simulink model "KR3_Modell"  (R2020a)
settings: Solver=VariableStepAuto  StartTime=0.0  StopTime=10.0  FixedStep=0.001  RelTol=1e-3
model workspace (MAT data in the model file):
  Damping = 0.2
  H = 2
  KR3_rbt = robotics.RigidBodyTree
  KR3_rbt.TreeInternal = robotics.manip.internal.RigidBodyTree
  KR3_rbt.TreeInternal.NumBodies = 6
  KR3_rbt.TreeInternal.Base = robotics.manip.internal.RigidBody
  KR3_rbt.TreeInternal.Base.Index = 0
  KR3_rbt.TreeInternal.Base.NameInternal = 'base'
  KR3_rbt.TreeInternal.Base.JointInternal = robotics.Joint
  KR3_rbt.TreeInternal.Base.JointInternal.Type = 'fixed'
  KR3_rbt.TreeInternal.Base.JointInternal.VelocityNumber = 0
  KR3_rbt.TreeInternal.Base.JointInternal.PositionNumber = 0
  KR3_rbt.TreeInternal.Base.JointInternal.MotionSubspace = [0; 0; 0; 0; 0; 0]
  KR3_rbt.TreeInternal.Base.JointInternal.NameInternal = 'base_jnt'
  KR3_rbt.TreeInternal.Base.ParentIndex = -1
  KR3_rbt.TreeInternal.Base.ChildrenIndices = 1
  KR3_rbt.TreeInternal.Base.MassInternal = 1
  KR3_rbt.TreeInternal.Base.CenterOfMassInternal = [0 0 0]
  KR3_rbt.TreeInternal.Base.InertiaInternal = [1  0  0; 0  1  0; 0  0  1]
  KR3_rbt.TreeInternal.Base.SpatialInertia = [1  0  0  0  0  0; 0  1  0  0  0  0; 0  0  1  0  0  0; 0  0  0  1  0  0; 0  0  0  0  1  0; 0  0  0  0  0  1]
  KR3_rbt.TreeInternal.Base.VisualsInternal{1} = robotics.manip.internal.RigidBodyGeometry
  KR3_rbt.TreeInternal.Base.VisualsInternal{1}.SourceData = {'Mesh', 'D:\Studium\SoSe21\MA_Arbeit\CAD-Dateien\baseMesh.stl'}
  KR3_rbt.TreeInternal.Base.VisualsInternal{1}.Vertices = [-0.0632426813245 -0.066875256598 -0.067146487534 -0.0603312700987 -0.0574519783258 -0.0620885789394 -0.0587106980383 -0.0573099479079 -0.052574519068 -0.0562280230224 -0.0555760525167 -0.0551131367683 ... (34239 elements, 11413x3)]
  KR3_rbt.TreeInternal.Base.VisualsInternal{1}.Faces = [1 4 7 8 8 10 11 12 13 16 16 20 ... (120618 elements, 40206x3)]
  KR3_rbt.TreeInternal.Base.CollisionsInternal = robotics.manip.internal.CollisionSet
  KR3_rbt.TreeInternal.Base.CollisionsInternal.MaxElements = 0
  KR3_rbt.TreeInternal.FastVisualizationHelper = robotics.manip.internal.FastVisualizationHelper
  KR3_rbt.TreeInternal.FastVisualizationHelper.IsUpdated = 0
  KR3_rbt.TreeInternal.FastVisualizationHelper.MeshAndFrameOptions = [0 1 1]
  KR3_rbt.TreeInternal.Gravity = [0 0 -9.80665]
  KR3_rbt.TreeInternal.Bodies{1} = robotics.manip.internal.RigidBody
  KR3_rbt.TreeInternal.Bodies{1}.Index = 1
  KR3_rbt.TreeInternal.Bodies{1}.NameInternal = 'body1'
  KR3_rbt.TreeInternal.Bodies{1}.JointInternal = robotics.Joint
  KR3_rbt.TreeInternal.Bodies{1}.JointInternal.Type = 'revolute'
  KR3_rbt.TreeInternal.Bodies{1}.JointInternal.VelocityNumber = 1
  KR3_rbt.TreeInternal.Bodies{1}.JointInternal.PositionNumber = 1
  KR3_rbt.TreeInternal.Bodies{1}.JointInternal.MotionSubspace = [0; 0; 1; 0; 0; 0]
  KR3_rbt.TreeInternal.Bodies{1}.JointInternal.InTree = 1
  KR3_rbt.TreeInternal.Bodies{1}.JointInternal.JointToParentTransform = [1  0  0  0; 0  -1  -1.22464679915e-16  0; 0  1.22464679915e-16  -1  0.183; 0  0  0  1]
  KR3_rbt.TreeInternal.Bodies{1}.JointInternal.NameInternal = 'jnt1'
  KR3_rbt.TreeInternal.Bodies{1}.JointInternal.PositionLimitsInternal = [-2.96705972839 2.96705972839]
  KR3_rbt.TreeInternal.Bodies{1}.JointInternal.JointAxisInternal = [0 0 1]
  KR3_rbt.TreeInternal.Bodies{1}.ParentIndex = 0
  KR3_rbt.TreeInternal.Bodies{1}.ChildrenIndices = [0 1]
  KR3_rbt.TreeInternal.Bodies{1}.MassInternal = 1
  KR3_rbt.TreeInternal.Bodies{1}.CenterOfMassInternal = [0 0 0]
  KR3_rbt.TreeInternal.Bodies{1}.InertiaInternal = [1  0  0; 0  1  0; 0  0  1]
  KR3_rbt.TreeInternal.Bodies{1}.SpatialInertia = [1  0  0  0  0  0; 0  1  0  0  0  0; 0  0  1  0  0  0; 0  0  0  1  0  0; 0  0  0  0  1  0; 0  0  0  0  0  1]
  KR3_rbt.TreeInternal.Bodies{1}.VisualsInternal{1} = robotics.manip.internal.RigidBodyGeometry
  KR3_rbt.TreeInternal.Bodies{1}.VisualsInternal{1}.SourceData = {'Mesh', 'D:\Studium\SoSe21\MA_Arbeit\CAD-Dateien\body1Mesh.stl'}
  KR3_rbt.TreeInternal.Bodies{1}.VisualsInternal{1}.Vertices = [0.010199774988 0.00763257872313 0.00765040656552 0.00609336374328 0.00559485983104 0.00148052396253 0.00461691664532 0.00193680962548 0.0066404142417 0.00471198977903 0.0110220154747 0.0100443195552 ... (42369 elements, 14123x3)]
  KR3_rbt.TreeInternal.Bodies{1}.VisualsInternal{1}.Faces = [1 2 3 6 5 4 4 1 2 9 7 11 ... (84738 elements, 28246x3)]
  KR3_rbt.TreeInternal.Bodies{1}.VisualsInternal{1}.Tform = [1  0  0  0; 0  -1  -1.22464679915e-16  0; 0  1.22464679915e-16  -1  0.183; 0  0  0  1]
  KR3_rbt.TreeInternal.Bodies{1}.CollisionsInternal = robotics.manip.internal.CollisionSet
  KR3_rbt.TreeInternal.Bodies{1}.CollisionsInternal.MaxElements = 0
  KR3_rbt.TreeInternal.Bodies{2} = robotics.manip.internal.RigidBody
  KR3_rbt.TreeInternal.Bodies{2}.Index = 2
  KR3_rbt.TreeInternal.Bodies{2}.NameInternal = 'body2'
  KR3_rbt.TreeInternal.Bodies{2}.JointInternal = robotics.Joint
  KR3_rbt.TreeInternal.Bodies{2}.JointInternal.Type = 'revolute'
  KR3_rbt.TreeInternal.Bodies{2}.JointInternal.VelocityNumber = 1
  KR3_rbt.TreeInternal.Bodies{2}.JointInternal.PositionNumber = 1
  KR3_rbt.TreeInternal.Bodies{2}.JointInternal.MotionSubspace = [0; 0; 1; 0; 0; 0]
  KR3_rbt.TreeInternal.Bodies{2}.JointInternal.InTree = 1
  KR3_rbt.TreeInternal.Bodies{2}.JointInternal.JointToParentTransform = [1  0  0  0.02; 0  6.12323399574e-17  -1  0; 0  1  6.12323399574e-17  -0.162; 0  0  0  1]
  KR3_rbt.TreeInternal.Bodies{2}.JointInternal.NameInternal = 'jnt2'
  KR3_rbt.TreeInternal.Bodies{2}.JointInternal.PositionLimitsInternal = [-2.96705972839 0.872664625997]
  KR3_rbt.TreeInternal.Bodies{2}.JointInternal.HomePositionInternal = -1.57079632679
  KR3_rbt.TreeInternal.Bodies{2}.JointInternal.JointAxisInternal = [0 0 1]
  KR3_rbt.TreeInternal.Bodies{2}.ParentIndex = 1
  KR3_rbt.TreeInternal.Bodies{2}.ChildrenIndices = [0 0 1]
  KR3_rbt.TreeInternal.Bodies{2}.MassInternal = 1
  KR3_rbt.TreeInternal.Bodies{2}.CenterOfMassInternal = [0 0 0]
  KR3_rbt.TreeInternal.Bodies{2}.InertiaInternal = [1  0  0; 0  1  0; 0  0  1]
  KR3_rbt.TreeInternal.Bodies{2}.SpatialInertia = [1  0  0  0  0  0; 0  1  0  0  0  0; 0  0  1  0  0  0; 0  0  0  1  0  0; 0  0  0  0  1  0; 0  0  0  0  0  1]
  KR3_rbt.TreeInternal.Bodies{2}.VisualsInternal{1} = robotics.manip.internal.RigidBodyGeometry
  KR3_rbt.TreeInternal.Bodies{2}.VisualsInternal{1}.SourceData = {'Mesh', 'D:\Studium\SoSe21\MA_Arbeit\CAD-Dateien\body2Mesh.stl'}
  KR3_rbt.TreeInternal.Bodies{2}.VisualsInternal{1}.Vertices = [0.0538231767714 0.0502161644399 0.0487190485001 0.0545652471483 0.044657304883 0.0434569939971 0.0580009557307 0.0581144578755 0.0390208996832 0.037002377212 0.0611467398703 0.0610443204641 ... (29349 elements, 9783x3)]
  KR3_rbt.TreeInternal.Bodies{2}.VisualsInternal{1}.Faces = [1 1 2 3 1 7 5 9 7 11 9 13 ... (58686 elements, 19562x3)]
  KR3_rbt.TreeInternal.Bodies{2}.VisualsInternal{1}.Tform = [6.12323399574e-17  1.83697019872e-16  1  -0.345; 1  -1.124819837e-32  -6.12323399574e-17  -0.02; 3.03535178041e-49  1  -1.83697019872e-16  4.35361937097e-17; 0  0  0  1]
  KR3_rbt.TreeInternal.Bodies{2}.CollisionsInternal = robotics.manip.internal.CollisionSet
  KR3_rbt.TreeInternal.Bodies{2}.CollisionsInternal.MaxElements = 0
  KR3_rbt.TreeInternal.Bodies{3} = robotics.manip.internal.RigidBody
  KR3_rbt.TreeInternal.Bodies{3}.Index = 3
  KR3_rbt.TreeInternal.Bodies{3}.NameInternal = 'body3'
  KR3_rbt.TreeInternal.Bodies{3}.JointInternal = robotics.Joint
  KR3_rbt.TreeInternal.Bodies{3}.JointInternal.Type = 'revolute'
  KR3_rbt.TreeInternal.Bodies{3}.JointInternal.VelocityNumber = 1
  KR3_rbt.TreeInternal.Bodies{3}.JointInternal.PositionNumber = 1
  KR3_rbt.TreeInternal.Bodies{3}.JointInternal.MotionSubspace = [0; 0; 1; 0; 0; 0]
  KR3_rbt.TreeInternal.Bodies{3}.JointInternal.InTree = 1
  KR3_rbt.TreeInternal.Bodies{3}.JointInternal.JointToParentTransform = [1  0  0  0.26; 0  1  0  0; 0  0  1  0; 0  0  0  1]
  KR3_rbt.TreeInternal.Bodies{3}.JointInternal.NameInternal = 'jnt3'
  KR3_rbt.TreeInternal.Bodies{3}.JointInternal.PositionLimitsInternal = [-1.91986217719 2.70526034059]
  KR3_rbt.TreeInternal.Bodies{3}.JointInternal.HomePositionInternal = 1.57079632679
  KR3_rbt.TreeInternal.Bodies{3}.JointInternal.JointAxisInternal = [0 0 1]
  KR3_rbt.TreeInternal.Bodies{3}.ParentIndex = 2
  KR3_rbt.TreeInternal.Bodies{3}.ChildrenIndices = [0 0 0 1]
  KR3_rbt.TreeInternal.Bodies{3}.MassInternal = 1
  KR3_rbt.TreeInternal.Bodies{3}.CenterOfMassInternal = [0 0 0]
  KR3_rbt.TreeInternal.Bodies{3}.InertiaInternal = [1  0  0; 0  1  0; 0  0  1]
  KR3_rbt.TreeInternal.Bodies{3}.SpatialInertia = [1  0  0  0  0  0; 0  1  0  0  0  0; 0  0  1  0  0  0; 0  0  0  1  0  0; 0  0  0  0  1  0; 0  0  0  0  0  1]
  KR3_rbt.TreeInternal.Bodies{3}.VisualsInternal{1} = robotics.manip.internal.RigidBodyGeometry
  KR3_rbt.TreeInternal.Bodies{3}.VisualsInternal{1}.SourceData = {'Mesh', 'D:\Studium\SoSe21\MA_Arbeit\CAD-Dateien\body3Mesh.stl'}
  KR3_rbt.TreeInternal.Bodies{3}.VisualsInternal{1}.Vertices = [0.130464464426 0.133762553334 0.129669874907 0.131500005722 0.132705897093 0.134124994278 0.133484452963 0.129170358181 0.13330963254 0.128999993205 0.134000003338 0.134547069669 ... (15924 elements, 5308x3)]
  KR3_rbt.TreeInternal.Bodies{3}.VisualsInternal{1}.Faces = [1 4 5 4 3 2 8 7 11 5 9 11 ... (31860 elements, 10620x3)]
  KR3_rbt.TreeInternal.Bodies{3}.VisualsInternal{1}.Tform = [1  0  0  -0.02; 0  -1.83697019872e-16  -1  0.605; 0  1  -1.83697019872e-16  4.35361937097e-17; 0  0  0  1]
  KR3_rbt.TreeInternal.Bodies{3}.CollisionsInternal = robotics.manip.internal.CollisionSet
  KR3_rbt.TreeInternal.Bodies{3}.CollisionsInternal.MaxElements = 0
  KR3_rbt.TreeInternal.Bodies{4} = robotics.manip.internal.RigidBody
  KR3_rbt.TreeInternal.Bodies{4}.Index = 4
  KR3_rbt.TreeInternal.Bodies{4}.NameInternal = 'body4'
  KR3_rbt.TreeInternal.Bodies{4}.JointInternal = robotics.Joint
  KR3_rbt.TreeInternal.Bodies{4}.JointInternal.Type = 'revolute'
  KR3_rbt.TreeInternal.Bodies{4}.JointInternal.VelocityNumber = 1
  KR3_rbt.TreeInternal.Bodies{4}.JointInternal.PositionNumber = 1
  KR3_rbt.TreeInternal.Bodies{4}.JointInternal.MotionSubspace = [0; 0; 1; 0; 0; 0]
  KR3_rbt.TreeInternal.Bodies{4}.JointInternal.InTree = 1
  KR3_rbt.TreeInternal.Bodies{4}.JointInternal.JointToParentTransform = [6.12323399574e-17  6.12323399574e-17  -1  0.122; -1  3.74939945665e-33  -6.12323399574e-17  -0.02; 0  1  6.12323399574e-17  0; 0  0  0  1]
  KR3_rbt.TreeInternal.Bodies{4}.JointInternal.NameInternal = 'jnt4'
  KR3_rbt.TreeInternal.Bodies{4}.JointInternal.PositionLimitsInternal = [-3.05432619099 3.05432619099]
  KR3_rbt.TreeInternal.Bodies{4}.JointInternal.JointAxisInternal = [0 0 1]
  KR3_rbt.TreeInternal.Bodies{4}.ParentIndex = 3
  KR3_rbt.TreeInternal.Bodies{4}.ChildrenIndices = [0 0 0 0 1]
  KR3_rbt.TreeInternal.Bodies{4}.MassInternal = 1
  KR3_rbt.TreeInternal.Bodies{4}.CenterOfMassInternal = [0 0 0]
  KR3_rbt.TreeInternal.Bodies{4}.InertiaInternal = [1  0  0; 0  1  0; 0  0  1]
  KR3_rbt.TreeInternal.Bodies{4}.SpatialInertia = [1  0  0  0  0  0; 0  1  0  0  0  0; 0  0  1  0  0  0; 0  0  0  1  0  0; 0  0  0  0  1  0; 0  0  0  0  0  1]
  KR3_rbt.TreeInternal.Bodies{4}.VisualsInternal{1} = robotics.manip.internal.RigidBodyGeometry
  KR3_rbt.TreeInternal.Bodies{4}.VisualsInternal{1}.SourceData = {'Mesh', 'D:\Studium\SoSe21\MA_Arbeit\CAD-Dateien\body4Mesh.stl'}
  KR3_rbt.TreeInternal.Bodies{4}.VisualsInternal{1}.Vertices = [0.2374278754 0.2374278754 0.2374278754 0.2374278754 0.237574264407 0.237607881427 0.237607881427 0.237574264407 0.237541690469 0.237541690469 0.237512126565 0.237512126565 ... (31293 elements, 10431x3)]
  KR3_rbt.TreeInternal.Bodies{4}.VisualsInternal{1}.Faces = [1 1 5 5 9 9 11 11 13 13 15 15 ... (62406 elements, 20802x3)]
  KR3_rbt.TreeInternal.Bodies{4}.VisualsInternal{1}.Tform = [6.12323399574e-17  1.83697019872e-16  1  -0.625; 6.12323399574e-17  1  -1.83697019872e-16  3.48412014357e-17; -1  6.12323399574e-17  6.12323399574e-17  0.142; 0  0  0  1]
  KR3_rbt.TreeInternal.Bodies{4}.CollisionsInternal = robotics.manip.internal.CollisionSet
  KR3_rbt.TreeInternal.Bodies{4}.CollisionsInternal.MaxElements = 0
  KR3_rbt.TreeInternal.Bodies{5} = robotics.manip.internal.RigidBody
  KR3_rbt.TreeInternal.Bodies{5}.Index = 5
  KR3_rbt.TreeInternal.Bodies{5}.NameInternal = 'body5'
  KR3_rbt.TreeInternal.Bodies{5}.JointInternal = robotics.Joint
  KR3_rbt.TreeInternal.Bodies{5}.JointInternal.Type = 'revolute'
  KR3_rbt.TreeInternal.Bodies{5}.JointInternal.VelocityNumber = 1
  KR3_rbt.TreeInternal.Bodies{5}.JointInternal.PositionNumber = 1
  KR3_rbt.TreeInternal.Bodies{5}.JointInternal.MotionSubspace = [0; 0; 1; 0; 0; 0]
  KR3_rbt.TreeInternal.Bodies{5}.JointInternal.InTree = 1
  KR3_rbt.TreeInternal.Bodies{5}.JointInternal.JointToParentTransform = [3.74939945665e-33  -1  6.12323399574e-17  0; 6.12323399574e-17  6.12323399574e-17  1  0; -1  0  6.12323399574e-17  -0.138; 0  0  0  1]
  KR3_rbt.TreeInternal.Bodies{5}.JointInternal.NameInternal = 'jnt5'
  KR3_rbt.TreeInternal.Bodies{5}.JointInternal.PositionLimitsInternal = [-2.09439510239 2.09439510239]
  KR3_rbt.TreeInternal.Bodies{5}.JointInternal.JointAxisInternal = [0 0 1]
  KR3_rbt.TreeInternal.Bodies{5}.ParentIndex = 4
  KR3_rbt.TreeInternal.Bodies{5}.ChildrenIndices = [0 0 0 0 0 1]
  KR3_rbt.TreeInternal.Bodies{5}.MassInternal = 1
  KR3_rbt.TreeInternal.Bodies{5}.CenterOfMassInternal = [0 0 0]
  KR3_rbt.TreeInternal.Bodies{5}.InertiaInternal = [1  0  0; 0  1  0; 0  0  1]
  KR3_rbt.TreeInternal.Bodies{5}.SpatialInertia = [1  0  0  0  0  0; 0  1  0  0  0  0; 0  0  1  0  0  0; 0  0  0  1  0  0; 0  0  0  0  1  0; 0  0  0  0  0  1]
  KR3_rbt.TreeInternal.Bodies{5}.VisualsInternal{1} = robotics.manip.internal.RigidBodyGeometry
  KR3_rbt.TreeInternal.Bodies{5}.VisualsInternal{1}.SourceData = {'Mesh', 'D:\Studium\SoSe21\MA_Arbeit\CAD-Dateien\body5Mesh.stl'}
  KR3_rbt.TreeInternal.Bodies{5}.VisualsInternal{1}.Vertices = [0.280791640282 0.280418545008 0.280028581619 0.281197071075 0.280991524458 0.281554192305 0.280000001192 0.280000001192 0.281901538372 0.281152635813 0.28150805831 0.280768126249 ... (183075 elements, 61025x3)]
  KR3_rbt.TreeInternal.Bodies{5}.VisualsInternal{1}.Faces = [1 4 6 2 3 2 5 9 11 13 10 14 ... (366135 elements, 122045x3)]
  KR3_rbt.TreeInternal.Bodies{5}.VisualsInternal{1}.Tform = [1  -7.49879891331e-33  -6.12323399574e-17  -0.28; -6.12323399574e-17  -1.22464679915e-16  -1  0.625; 4.82715273077e-33  1  -1.22464679915e-16  1.37160441505e-17; 0  0  0  1]
  KR3_rbt.TreeInternal.Bodies{5}.CollisionsInternal = robotics.manip.internal.CollisionSet
  KR3_rbt.TreeInternal.Bodies{5}.CollisionsInternal.MaxElements = 0
  KR3_rbt.TreeInternal.Bodies{6} = robotics.manip.internal.RigidBody
  KR3_rbt.TreeInternal.Bodies{6}.Index = 6
  KR3_rbt.TreeInternal.Bodies{6}.NameInternal = 'body6'
  KR3_rbt.TreeInternal.Bodies{6}.JointInternal = robotics.Joint
  KR3_rbt.TreeInternal.Bodies{6}.JointInternal.Type = 'revolute'
  KR3_rbt.TreeInternal.Bodies{6}.JointInternal.VelocityNumber = 1
  KR3_rbt.TreeInternal.Bodies{6}.JointInternal.PositionNumber = 1
  KR3_rbt.TreeInternal.Bodies{6}.JointInternal.MotionSubspace = [0; 0; 1; 0; 0; 0]
  KR3_rbt.TreeInternal.Bodies{6}.JointInternal.InTree = 1
  KR3_rbt.TreeInternal.Bodies{6}.JointInternal.JointToParentTransform = [6.12323399574e-17  6.12323399574e-17  -1  0.075; -1  3.74939945665e-33  -6.12323399574e-17  0; 0  1  6.12323399574e-17  0; 0  0  0  1]
  KR3_rbt.TreeInternal.Bodies{6}.JointInternal.NameInternal = 'jnt6'
  KR3_rbt.TreeInternal.Bodies{6}.JointInternal.PositionLimitsInternal = [-6.10865238198 6.10865238198]
  KR3_rbt.TreeInternal.Bodies{6}.JointInternal.JointAxisInternal = [0 0 1]
  KR3_rbt.TreeInternal.Bodies{6}.ParentIndex = 5
  KR3_rbt.TreeInternal.Bodies{6}.ChildrenIndices = [0 0 0 0 0]
  KR3_rbt.TreeInternal.Bodies{6}.MassInternal = 1
  KR3_rbt.TreeInternal.Bodies{6}.CenterOfMassInternal = [0 0 0]
  KR3_rbt.TreeInternal.Bodies{6}.InertiaInternal = [1  0  0; 0  1  0; 0  0  1]
  KR3_rbt.TreeInternal.Bodies{6}.SpatialInertia = [1  0  0  0  0  0; 0  1  0  0  0  0; 0  0  1  0  0  0; 0  0  0  1  0  0; 0  0  0  0  1  0; 0  0  0  0  0  1]
  KR3_rbt.TreeInternal.Bodies{6}.VisualsInternal{1} = robotics.manip.internal.RigidBodyGeometry
  KR3_rbt.TreeInternal.Bodies{6}.VisualsInternal{1}.SourceData = {'Mesh', 'D:\Studium\SoSe21\MA_Arbeit\CAD-Dateien\body6Mesh.stl'}
  KR3_rbt.TreeInternal.Bodies{6}.VisualsInternal{1}.Vertices = [0.338999986649 0.338999986649 0.338999986649 0.338999986649 0.338999986649 0.338999986649 0.338999986649 0.338999986649 0.338999986649 0.338999986649 0.338999986649 0.338999986649 ... (7587 elements, 2529x3)]
  KR3_rbt.TreeInternal.Bodies{6}.VisualsInternal{1}.Faces = [1 4 4 6 7 8 8 10 11 11 13 14 ... (15174 elements, 5058x3)]
  KR3_rbt.TreeInternal.Bodies{6}.VisualsInternal{1}.Tform = [1.22464679915e-16  1.22464679915e-16  1  -0.625; 6.12323399574e-17  1  -1.22464679915e-16  -8.02143653442e-18; -1  6.12323399574e-17  1.22464679915e-16  0.355; 0  0  0  1]
  KR3_rbt.TreeInternal.Bodies{6}.CollisionsInternal = robotics.manip.internal.CollisionSet
  KR3_rbt.TreeInternal.Bodies{6}.CollisionsInternal.MaxElements = 0
  KR3_rbt.TreeInternal.NumNonFixedBodies = 6
  KR3_rbt.TreeInternal.PositionNumber = 6
  KR3_rbt.TreeInternal.VelocityNumber = 6
  KR3_rbt.TreeInternal.PositionDoFMap = [1  1; 2  2; 3  3; 4  4; 5  5; 6  6]
  KR3_rbt.TreeInternal.VelocityDoFMap = [1  1; 2  2; 3  3; 4  4; 5  5; 6  6]
  KR3_rbt.TreeInternal.MaxNumBodies = 6
  KR3_rbt.TreeInternal.MaxNameLength = 200
  KR3_rbt.TreeInternal.MaxJointPositionNumber = 7
  KR3_rbt.TreeInternal.VisualizationInfo = robotics.manip.internal.VisualizationInfo
  KR3_rbt.TreeInternal.VisualizationInfo.ShowTag = 'DO_NOT_EDIT_41EHK'
  KR3_rbt.TreeInternal.DataFormatInternal = 'column'
  L = 20
  W = 2
  den = 1110
  initTargetPose = [0.264 0 0.61 -0.471238898038 1.32645023152 -0.418879020479]
  rho = 1000
  st = 0.04
  tol = 0.01
values from neighbouring files (symbols this model uses):
  s = char(posmsg{k})    [Messbahn_Quadrat.m]
  traj = [traj, axis_conf]    [generate_trajectory.m]
undefined symbols (not defined in the file or in its folder): X, Y, Z
libraries: sm_lib x33, nesl_utility x17, fl_ps_legacy_lib x12, simulink x1
settings Model: OrderedModelArguments=off  Creator=Arbeit  LastModifiedBy=Arbeit
settings DataIOCC: ReturnWorkspaceOutputs=off
settings DebuggingCC: ArithmeticOperatorsInVariantConditions=warning
settings SFSimCC: SimUseLocalCustomCode=off  CustomCodeUndefinedFunction=UseInterfaceOnly
settings RTWCC: RTWUseLocalCustomCode=off

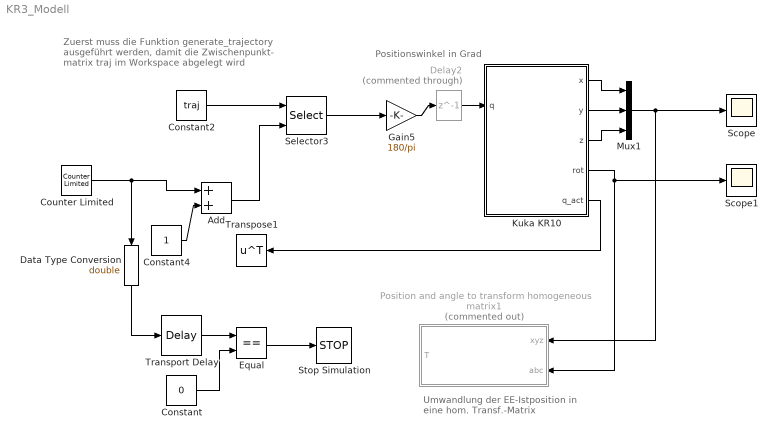
== system KR3_Modell ==
  note: Zuerst muss die Funktion generate_trajectory
      | ausgeführt werden, damit die Zwischenpunkt-
      | matrix traj im Workspace abgelegt wird
  note: Positionswinkel in Grad
  note: Umwandlung der EE-Istposition in eine hom. Transf.-Matrix
  Add : Sum
  Constant : Constant  Value=0
  Constant2 : Constant  Value=traj
  Constant4 : Constant
  Counter Limited : simulink/Sources/Counter Limited  uplimit=size(traj,2)-1  tsamp=-1
  Data Type Conversion : DataTypeConversion  OutDataTypeStr=double
  Delay2 : Delay  Commented=through  DelayLength=1
  Equal : RelationalOperator  Operator===  OutDataTypeStr=boolean  RndMeth=Simplest
  Gain5 : Gain  Gain=180/pi
  Kuka KR10 : Subsystem
      mask Display: image('kuka_kr10_r1100.jpg');
  Mux1 : Mux  Inputs=3
  Position and angle to transform homogeneous matrix1 : MATLAB Function  Commented=on  TreatAsAtomicUnit=on
  Scope : Scope
  Scope1 : Scope
  Selector3 : Selector  NumberOfDimensions=2  InputPortWidth=3  IndexOptions=Select all,Starting index (port)  Indices=[1 3],1  OutputSizes=1,1
  Stop Simulation : Stop
  Transport Delay : TransportDelay  InitialOutput=1
  Transpose1 : Math  Operator=transpose  SaturateOnIntegerOverflow=on
  wires:
  Kuka KR10/2(y) -> Mux1/2
  Kuka KR10/1(x) -> Mux1/1
  Kuka KR10/3(z) -> Mux1/3
  Kuka KR10/4(rot) -> Position and angle to transform homogeneous matrix1/2(abc), Scope1/1
  Mux1/1 -> Position and angle to transform homogeneous matrix1/1(xyz), Scope/1
  Constant2/1 -> Selector3/1
  Selector3/1 -> Gain5/1
  Gain5/1 -> Delay2/1
  Delay2/1 -> Kuka KR10/1(q)
  Kuka KR10/5(q_act) -> Transpose1/1
  Counter Limited/1 -> Add/1, Data Type Conversion/1
  Add/1 -> Selector3/2
  Constant4/1 -> Add/2
  Transport Delay/1 -> Equal/1
  Constant/1 -> Equal/2
  Equal/1 -> Stop Simulation/1
  Data Type Conversion/1 -> Transport Delay/1

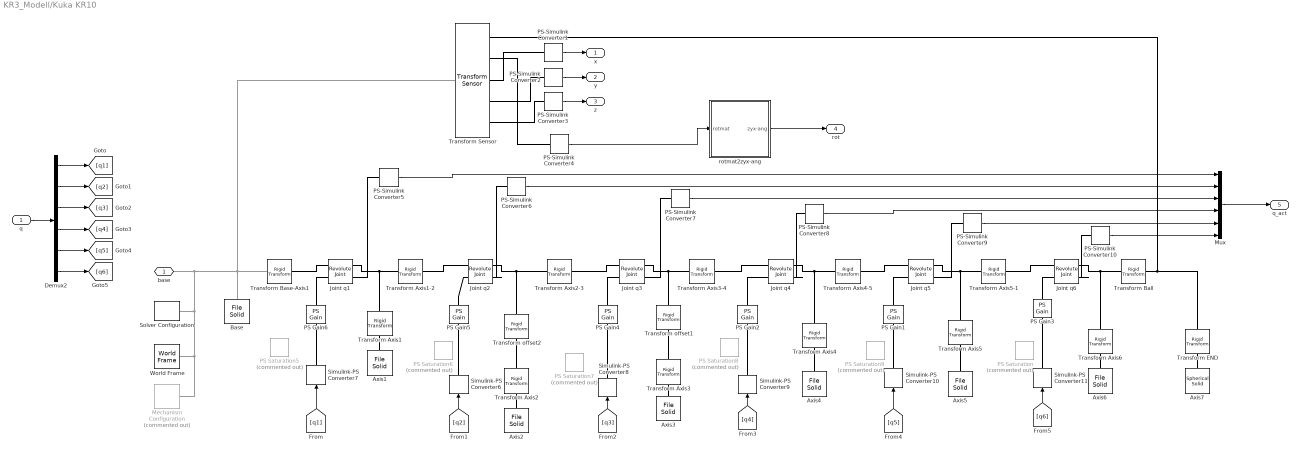
== system KR3_Modell/Kuka KR10 ==
  q : Inport
   Joint q{1..6} (6 alike) : sm_lib/Joints/Revolute Joint  JointMode=Normal  SenseConstraintForce=off  SenseConstraintForceX=off  SenseConstraintForceY=off  SenseConstraintForceZ=off  SenseConstraintTorque=off  SenseConstraintTorqueX=off  SenseConstraintTorqueY=off  SenseConstraintTorqueZ=off  SenseTotalForce=off  SenseTotalForceX=off  SenseTotalForceY=off  SenseTotalForceZ=off  SenseTotalTorque=off  SenseTotalTorqueX=off  SenseTotalTorqueY=off  SenseTotalTorqueZ=off  CompositeWrenchDir=FollowerOnBase  CompositeWrenchFrame=BaseFrame  EquilibriumPosition=0  EquilibriumPositionUnits=deg  SpringStiffness=0  SpringStiffnessUnits=N*m/deg  DampingCoefficient=0  DampingCoefficientUnits=N*m/(deg/s)  TorqueActuationMode=ComputedTorque  MotionActuationMode=InputMotion  SensePosition=on  SenseVelocity=off  SenseAcceleration=off  SenseTorqueForce=off  SenseLowerLimitTorqueForce=off  SenseUpperLimitTorqueForce=off  LowerLimitSpecify=off  LowerLimitBound=-90  LowerLimitBoundUnits=deg  LowerLimitStiffness=1e4  LowerLimitStiffnessUnits=N*m/deg  LowerLimitDamping=10  LowerLimitDampingUnits=N*m/(deg/s)  LowerLimitTransitionRegionWidth=0.1  LowerLimitTransitionRegionWidthUnits=deg  UpperLimitSpecify=off  UpperLimitBound=90  UpperLimitBoundUnits=deg  UpperLimitStiffness=1e4  UpperLimitStiffnessUnits=N*m/deg  UpperLimitDamping=10  UpperLimitDampingUnits=N*m/(deg/s)  UpperLimitTransitionRegionWidth=0.1  UpperLimitTransitionRegionWidthUnits=deg  PositionTargetSpecify=on  PositionTargetPriority=Low  PositionTargetValue=0  PositionTargetValueUnits=deg  VelocityTargetSpecify=off  VelocityTargetPriority=High  VelocityTargetValue=0  VelocityTargetValueUnits=deg/s
  Axis1 : sm_lib/Body Elements/File Solid  ExtGeomFileName=D:\Studium\SoSe21\MA_Arbeit\CAD-Dateien\body1Test.step  UnitType=FromFile  ExtGeomFileUnits=m  StepReaderType=OCC  ExportConvexHullGeometry=off  InertiaType=CalculateFromGeometry  Mass=1  MassUnits=kg  CenterOfMass=[0 0 0]  CenterOfMassUnits=m  MomentsOfInertia=[1 1 1]  MomentsOfInertiaUnits=kg*m^2  ProductsOfInertia=[1 1 1]  ProductsOfInertiaUnits=kg*m^2  BasedOnType=Density  Density=den  DensityUnits=kg/m^3  DoExposeReferenceFrame=on  SerializedFrames=<Frames/>  GraphicType=FromGeometry  MarkerShape=Sphere  MarkerSize=10  GraphicVisPropType=SimpleVisualProperties  GraphicDiffuseColor=[1 0.39 0]  GraphicSpecularColor=[0.5 0.5 0.5 1.0]  GraphicAmbientColor=[0.15 0.15 0.15 1.0]  GraphicEmissiveColor=[0.0 0.0 0.0 1.0]  GraphicShininess=75  GraphicOpacity=1
  Axis2 : sm_lib/Body Elements/File Solid  ExtGeomFileName=D:\Studium\SoSe21\MA_Arbeit\CAD-Dateien\body2Test.step  UnitType=FromFile  ExtGeomFileUnits=m  StepReaderType=OCC  ExportConvexHullGeometry=off  InertiaType=CalculateFromGeometry  Mass=1  MassUnits=kg  CenterOfMass=[0 0 0]  CenterOfMassUnits=m  MomentsOfInertia=[1 1 1]  MomentsOfInertiaUnits=kg*m^2  ProductsOfInertia=[1 1 1]  ProductsOfInertiaUnits=kg*m^2  BasedOnType=Density  Density=den  DensityUnits=kg/m^3  DoExposeReferenceFrame=on  SerializedFrames=<Frames/>  GraphicType=FromGeometry  MarkerShape=Sphere  MarkerSize=10  GraphicVisPropType=SimpleVisualProperties  GraphicDiffuseColor=[1 0.39 0]  GraphicSpecularColor=[0.5 0.5 0.5 1.0]  GraphicAmbientColor=[0.15 0.15 0.15 1.0]  GraphicEmissiveColor=[0.0 0.0 0.0 1.0]  GraphicShininess=75  GraphicOpacity=1
  Axis3 : sm_lib/Body Elements/File Solid  ExtGeomFileName=D:\Studium\SoSe21\MA_Arbeit\CAD-Dateien\body3Test.step  UnitType=FromFile  ExtGeomFileUnits=m  StepReaderType=OCC  ExportConvexHullGeometry=off  InertiaType=CalculateFromGeometry  Mass=1  MassUnits=kg  CenterOfMass=[0 0 0]  CenterOfMassUnits=m  MomentsOfInertia=[1 1 1]  MomentsOfInertiaUnits=kg*m^2  ProductsOfInertia=[1 1 1]  ProductsOfInertiaUnits=kg*m^2  BasedOnType=Density  Density=den  DensityUnits=kg/m^3  DoExposeReferenceFrame=on  SerializedFrames=<Frames/>  GraphicType=FromGeometry  MarkerShape=Sphere  MarkerSize=10  GraphicVisPropType=SimpleVisualProperties  GraphicDiffuseColor=[1 0.39 0]  GraphicSpecularColor=[0.5 0.5 0.5 1.0]  GraphicAmbientColor=[0.15 0.15 0.15 1.0]  GraphicEmissiveColor=[0.0 0.0 0.0 1.0]  GraphicShininess=75  GraphicOpacity=1
  Axis4 : sm_lib/Body Elements/File Solid  ExtGeomFileName=D:\Studium\SoSe21\MA_Arbeit\CAD-Dateien\body4Test.step  UnitType=FromFile  ExtGeomFileUnits=m  StepReaderType=OCC  ExportConvexHullGeometry=off  InertiaType=CalculateFromGeometry  Mass=1  MassUnits=kg  CenterOfMass=[0 0 0]  CenterOfMassUnits=m  MomentsOfInertia=[1 1 1]  MomentsOfInertiaUnits=kg*m^2  ProductsOfInertia=[1 1 1]  ProductsOfInertiaUnits=kg*m^2  BasedOnType=Density  Density=den  DensityUnits=kg/m^3  DoExposeReferenceFrame=on  SerializedFrames=<Frames/>  GraphicType=FromGeometry  MarkerShape=Sphere  MarkerSize=10  GraphicVisPropType=SimpleVisualProperties  GraphicDiffuseColor=[1 0.39 0]  GraphicSpecularColor=[0.5 0.5 0.5 1.0]  GraphicAmbientColor=[0.15 0.15 0.15 1.0]  GraphicEmissiveColor=[0.0 0.0 0.0 1.0]  GraphicShininess=75  GraphicOpacity=1
  Axis5 : sm_lib/Body Elements/File Solid  ExtGeomFileName=D:\Studium\SoSe21\MA_Arbeit\CAD-Dateien\body5Test.step  UnitType=FromFile  ExtGeomFileUnits=m  StepReaderType=OCC  ExportConvexHullGeometry=off  InertiaType=CalculateFromGeometry  Mass=1  MassUnits=kg  CenterOfMass=[0 0 0]  CenterOfMassUnits=m  MomentsOfInertia=[1 1 1]  MomentsOfInertiaUnits=kg*m^2  ProductsOfInertia=[1 1 1]  ProductsOfInertiaUnits=kg*m^2  BasedOnType=Density  Density=den  DensityUnits=kg/m^3  DoExposeReferenceFrame=on  SerializedFrames=<Frames/>  GraphicType=FromGeometry  MarkerShape=Sphere  MarkerSize=10  GraphicVisPropType=SimpleVisualProperties  GraphicDiffuseColor=[1 0.39 0]  GraphicSpecularColor=[0.5 0.5 0.5 1.0]  GraphicAmbientColor=[0.15 0.15 0.15 1.0]  GraphicEmissiveColor=[0.0 0.0 0.0 1.0]  GraphicShininess=75  GraphicOpacity=1
  Axis6 : sm_lib/Body Elements/File Solid  ExtGeomFileName=D:\Studium\SoSe21\MA_Arbeit\CAD-Dateien\body6Test.step  UnitType=FromFile  ExtGeomFileUnits=m  StepReaderType=OCC  ExportConvexHullGeometry=off  InertiaType=CalculateFromGeometry  Mass=1  MassUnits=kg  CenterOfMass=[0 0 0]  CenterOfMassUnits=m  MomentsOfInertia=[1 1 1]  MomentsOfInertiaUnits=kg*m^2  ProductsOfInertia=[1 1 1]  ProductsOfInertiaUnits=kg*m^2  BasedOnType=Density  Density=den  DensityUnits=kg/m^3  DoExposeReferenceFrame=on  SerializedFrames=<Frames/>  GraphicType=FromGeometry  MarkerShape=Sphere  MarkerSize=10  GraphicVisPropType=SimpleVisualProperties  GraphicDiffuseColor=[.2 .2 .2]  GraphicSpecularColor=[0.5 0.5 0.5 1.0]  GraphicAmbientColor=[0.15 0.15 0.15 1.0]  GraphicEmissiveColor=[0.0 0.0 0.0 1.0]  GraphicShininess=75  GraphicOpacity=1
  Axis7 : sm_lib/Body Elements/Spherical Solid  GraphicAmbientColor=[0.15 0.15 0.15 1.0]  BasedOnType=Mass  CenterOfMass=[0 0 0]  CenterOfMassUnits=m  GraphicDiffuseColor=[1 1 1]  Density=den  DensityUnits=kg/m^3  DoExposeReferenceFrame=on  GraphicEmissiveColor=[0.0 0.0 0.0 1.0]  ExportEntireGeometry=off  SerializedExposedGeometries=<ExposedGeometries/>  SerializedFrames=<Frames/>  MarkerShape=Sphere  MarkerSize=10  GraphicType=FromGeometry  InertiaType=CalculateFromGeometry  Mass=0.254  MassUnits=kg  MomentsOfInertia=[1 1 1]  MomentsOfInertiaUnits=kg*m^2  GraphicOpacity=1  ProductsOfInertia=[1 1 1]  ProductsOfInertiaUnits=kg*m^2  GraphicShininess=75  GraphicSpecularColor=[0.5 0.5 0.5 1.0]  SphereRadius=0.034  SphereRadiusUnits=m  GraphicVisPropType=SimpleVisualProperties
  Base : sm_lib/Body Elements/File Solid  ExtGeomFileName=D:\Studium\SoSe21\MA_Arbeit\CAD-Dateien\baseTest.step  UnitType=FromFile  ExtGeomFileUnits=m  StepReaderType=OCC  ExportConvexHullGeometry=off  InertiaType=CalculateFromGeometry  Mass=1  MassUnits=kg  CenterOfMass=[0 0 0]  CenterOfMassUnits=m  MomentsOfInertia=[1 1 1]  MomentsOfInertiaUnits=kg*m^2  ProductsOfInertia=[1 1 1]  ProductsOfInertiaUnits=kg*m^2  BasedOnType=Density  Density=den  DensityUnits=kg/m^3  DoExposeReferenceFrame=on  SerializedFrames=<Frames/>  GraphicType=FromGeometry  MarkerShape=Sphere  MarkerSize=10  GraphicVisPropType=SimpleVisualProperties  GraphicDiffuseColor=[.2 .2 .2]  GraphicSpecularColor=[0.5 0.5 0.5 1.0]  GraphicAmbientColor=[0.15 0.15 0.15 1.0]  GraphicEmissiveColor=[0.0 0.0 0.0 1.0]  GraphicShininess=75  GraphicOpacity=1
  Demux2 : Demux  Outputs=6
  Mechanism Configuration : sm_lib/Utilities/Mechanism Configuration  Commented=on  UniformGravity=Constant  GravityVector=[0 0 -9.80665]  GravityVectorUnits=m/s^2  GravityUnits=m/s^2  LinearizationDelta=0.001  JointModeTransitionNonlinearIterations=2
  Mux : Mux  Inputs=6
  PS Gain{1..6} (6 alike) : fl_ps_legacy_lib/Legacy Physical Signals/Functions/PS Gain  gain=pi/180
  PS Saturation : fl_ps_legacy_lib/Legacy Physical Signals/Nonlinear Operators/PS Saturation  Commented=on  upper_limit=350  lower_limit=-350
      settings: SourceProductBaseCode=SS  InternalSimscapePortConfiguration="{\"Bottom\":[],\"Left\":[{\"id\":\"I\",\"label\":\"\",\"type\":\"input\"}],\"Right\":[{\"id\":\"O\",\"label\":\"\",\"type\":\"output\"}],\"Top\":[]}"
  PS Saturation5 : fl_ps_legacy_lib/Legacy Physical Signals/Nonlinear Operators/PS Saturation  Commented=on  upper_limit=170  lower_limit=-170
      settings: SourceProductBaseCode=SS  InternalSimscapePortConfiguration="{\"Bottom\":[],\"Left\":[{\"id\":\"I\",\"label\":\"\",\"type\":\"input\"}],\"Right\":[{\"id\":\"O\",\"label\":\"\",\"type\":\"output\"}],\"Top\":[]}"
  PS Saturation6 : fl_ps_legacy_lib/Legacy Physical Signals/Nonlinear Operators/PS Saturation  Commented=on  upper_limit=50  lower_limit=-170
      settings: SourceProductBaseCode=SS  InternalSimscapePortConfiguration="{\"Bottom\":[],\"Left\":[{\"id\":\"I\",\"label\":\"\",\"type\":\"input\"}],\"Right\":[{\"id\":\"O\",\"label\":\"\",\"type\":\"output\"}],\"Top\":[]}"
  PS Saturation7 : fl_ps_legacy_lib/Legacy Physical Signals/Nonlinear Operators/PS Saturation  Commented=on  upper_limit=155  lower_limit=-110
      settings: SourceProductBaseCode=SS  InternalSimscapePortConfiguration="{\"Bottom\":[],\"Left\":[{\"id\":\"I\",\"label\":\"\",\"type\":\"input\"}],\"Right\":[{\"id\":\"O\",\"label\":\"\",\"type\":\"output\"}],\"Top\":[]}"
  PS Saturation8 : fl_ps_legacy_lib/Legacy Physical Signals/Nonlinear Operators/PS Saturation  Commented=on  upper_limit=175  lower_limit=-175
      settings: SourceProductBaseCode=SS  InternalSimscapePortConfiguration="{\"Bottom\":[],\"Left\":[{\"id\":\"I\",\"label\":\"\",\"type\":\"input\"}],\"Right\":[{\"id\":\"O\",\"label\":\"\",\"type\":\"output\"}],\"Top\":[]}"
  PS Saturation9 : fl_ps_legacy_lib/Legacy Physical Signals/Nonlinear Operators/PS Saturation  Commented=on  upper_limit=120  lower_limit=-120
      settings: SourceProductBaseCode=SS  InternalSimscapePortConfiguration="{\"Bottom\":[],\"Left\":[{\"id\":\"I\",\"label\":\"\",\"type\":\"input\"}],\"Right\":[{\"id\":\"O\",\"label\":\"\",\"type\":\"output\"}],\"Top\":[]}"
  PS-Simulink Converter{1..10} (10 alike) : nesl_utility/PS-Simulink Converter  PhysicalDomain=network_engine_domain  SubClassName=ps_output  LeftPortType=input  RightPortType=output  PseudoPeriodic=off  Frequencies=[]  Unit=1  AffineConversion=off
      settings: SourceProductBaseCode=PW,SS
  Simulink-PS Converter{6..11} (6 alike) : nesl_utility/Simulink-PS Converter  PhysicalDomain=network_engine_domain  SubClassName=ps_input  LeftPortType=input  RightPortType=output  PseudoPeriodic=off  Frequencies=[]  NoiseDistribution=none  NoiseParameters=[]  Unit=1  AffineConversion=off  FilteringAndDerivatives=provide  SimscapeFilterOrder=1  InputFilterTimeConstant=0.001  UdotUserProvided=0
      settings: SourceProductBaseCode=PW,SS
  Solver Configuration : nesl_utility/Solver Configuration  PhysicalDomain=network_engine_domain  SubClassName=solver  LeftPortType=input  RightPortType=generic  Tones=[]  Harmonics=[]  SimulateNoise=off  Profile=off  UseLocalSampling=off  EnableSwitchedLinearOptims=on  FrequencyDomain=off  UseCCode=off  RelTol=0.001  AbsTol=1e-06  MinStep=1e-09  ToWorkspace=off  RevertToSquareIcSolve=off  NumHomotopyIterations=100  PhasorMode=off  PhasorModeNumHarmonics=1  DoDC=off  ResidualTolerance=1e-04  UseLocalSolver=on  LocalSolverChoice=NE_BACKWARD_EULER_ADVANCER  LocalSolverSampleTime=0.01  DoFixedCost=on  MaxNonlinIter=3  MaxModeIter=2  ComputeImpulses=off  ImpulseIterations=2  LinearAlgebra=auto  EquationFormulation=NE_TIME_EF  DelaysMemoryBudget=1024  AutomaticFiltering=on  FilteringTimeConstant=0.001  PartitionStorageMethod=AS_NEEDED  PartitionMemoryBudget=1024  PartitionMethod=FAST
      settings: SourceProductBaseCode=PW,SS
  Transform Sensor : sm_lib/Frames and Transforms/Transform Sensor  MeasurementFrame=World  SenseAngle=off  SenseAxis=off  SenseAngle1=off  SenseAngle2=off  SenseAngle3=off  SenseQ=off  SenseR=on  SenseOmegaX=off  SenseOmegaY=off  SenseOmegaZ=off  SenseOmega1=off  SenseOmega2=off  SenseOmega3=off  SenseQDot=off  SenseRDot=off  SenseAlphaX=off  SenseAlphaY=off  SenseAlphaZ=off  SenseAlpha1=off  SenseAlpha2=off  SenseAlpha3=off  SenseQDDot=off  SenseRDDot=off  SenseX=on  SenseY=on  SenseZ=on  SenseRad=off  SenseAzim=off  SenseDist=off  SenseInc=off  SenseXDot=off  SenseYDot=off  SenseZDot=off  SenseRadDot=off  SenseAzimDot=off  SenseDistDot=off  SenseIncDot=off  SenseXDDot=off  SenseYDDot=off  SenseZDDot=off  SenseRadDDot=off  SenseAzimDDot=off  SenseDistDDot=off  SenseIncDDot=off
  Transform Axis1 : sm_lib/Frames and Transforms/Rigid Transform  TranslationMethod=Cartesian  TranslationStandardOffset=0  TranslationLengthUnit=mm  TranslationStandardAxis=+Z  TranslationCartesianOffset=[0 0 183]  TranslationROffset=0  TranslationROffsetUnits=m  TranslationZOffset=0  TranslationZOffsetUnits=m  TranslationThetaOffset=0  TranslationThetaOffsetUnits=deg  RotationMethod=RotationSequence  RotationAngleUnits=deg  RotationStandardAxis=+Z  RotationAngle=0.0  RotationArbitraryAxis=[0 0 1]  FollAlignAxisA=+Z  BaseAlignAxisA=+Z  FollAlignAxisB=+X  BaseAlignAxisB=+X  RotationSequenceAxes=FollowerAxes  RotationSequence=ZYX  RotationSequenceAngles=[0 0 pi]  RotationSequenceAnglesUnits=rad  RotationMatrix=[1 0 0; 0 1 0; 0 0 1]
  Transform Axis1-2 : sm_lib/Frames and Transforms/Rigid Transform  TranslationMethod=Cartesian  TranslationStandardOffset=0  TranslationLengthUnit=mm  TranslationStandardAxis=+Z  TranslationCartesianOffset=[20 0 -162]  TranslationROffset=0  TranslationROffsetUnits=m  TranslationZOffset=0  TranslationZOffsetUnits=m  TranslationThetaOffset=0  TranslationThetaOffsetUnits=deg  RotationMethod=RotationSequence  RotationAngleUnits=deg  RotationStandardAxis=+Z  RotationAngle=0.0  RotationArbitraryAxis=[0 0 1]  FollAlignAxisA=+X  BaseAlignAxisA=+X  FollAlignAxisB=+Z  BaseAlignAxisB=-Y  RotationSequenceAxes=FollowerAxes  RotationSequence=ZYX  RotationSequenceAngles=[0 0 pi/2]  RotationSequenceAnglesUnits=rad  RotationMatrix=[1 0 0; 0 1 0; 0 0 1]
  Transform Axis2 : sm_lib/Frames and Transforms/Rigid Transform  TranslationMethod=Cartesian  TranslationStandardOffset=0  TranslationLengthUnit=mm  TranslationStandardAxis=+Z  TranslationCartesianOffset=[20 0 345]  TranslationROffset=0  TranslationROffsetUnits=m  TranslationZOffset=0  TranslationZOffsetUnits=m  TranslationThetaOffset=0  TranslationThetaOffsetUnits=deg  RotationMethod=RotationSequence  RotationAngleUnits=deg  RotationStandardAxis=-X  RotationAngle=90  RotationArbitraryAxis=[0 0 1]  FollAlignAxisA=+Z  BaseAlignAxisA=-Y  FollAlignAxisB=+X  BaseAlignAxisB=+X  RotationSequenceAxes=FollowerAxes  RotationSequence=ZYX  RotationSequenceAngles=[0 0 -90]  RotationSequenceAnglesUnits=deg  RotationMatrix=[1 0 0; 0 1 0; 0 0 1]
  Transform Axis2-3 : sm_lib/Frames and Transforms/Rigid Transform  TranslationMethod=Cartesian  TranslationStandardOffset=0  TranslationLengthUnit=mm  TranslationStandardAxis=+Z  TranslationCartesianOffset=[260 0 0]  TranslationROffset=0  TranslationROffsetUnits=m  TranslationZOffset=0  TranslationZOffsetUnits=m  TranslationThetaOffset=0  TranslationThetaOffsetUnits=deg  RotationMethod=RotationSequence  RotationAngleUnits=deg  RotationStandardAxis=+Z  RotationAngle=0.0  RotationArbitraryAxis=[0 0 1]  FollAlignAxisA=+Z  BaseAlignAxisA=+Z  FollAlignAxisB=+X  BaseAlignAxisB=+Y  RotationSequenceAxes=FollowerAxes  RotationSequence=ZYX  RotationSequenceAngles=[0 0 0]  RotationSequenceAnglesUnits=deg  RotationMatrix=[1 0 0; 0 1 0; 0 0 1]
  Transform Axis3 : sm_lib/Frames and Transforms/Rigid Transform  TranslationMethod=Cartesian  TranslationStandardOffset=0  TranslationLengthUnit=mm  TranslationStandardAxis=+Z  TranslationCartesianOffset=[20 0 605]  TranslationROffset=0  TranslationROffsetUnits=m  TranslationZOffset=0  TranslationZOffsetUnits=m  TranslationThetaOffset=0  TranslationThetaOffsetUnits=deg  RotationMethod=RotationSequence  RotationAngleUnits=deg  RotationStandardAxis=+Z  RotationAngle=0.0  RotationArbitraryAxis=[0 0 1]  FollAlignAxisA=+Z  BaseAlignAxisA=-Y  FollAlignAxisB=+X  BaseAlignAxisB=+Z  RotationSequenceAxes=FollowerAxes  RotationSequence=ZYX  RotationSequenceAngles=[0 -90 -90]  RotationSequenceAnglesUnits=deg  RotationMatrix=[1 0 0; 0 1 0; 0 0 1]
  Transform Axis3-4 : sm_lib/Frames and Transforms/Rigid Transform  TranslationMethod=Cartesian  TranslationStandardOffset=0  TranslationLengthUnit=mm  TranslationStandardAxis=+Z  TranslationCartesianOffset="[122  -20  0]"  TranslationROffset=0  TranslationROffsetUnits=m  TranslationZOffset=0  TranslationZOffsetUnits=m  TranslationThetaOffset=0  TranslationThetaOffsetUnits=deg  RotationMethod=RotationSequence  RotationAngleUnits=deg  RotationStandardAxis=+Z  RotationAngle=0.0  RotationArbitraryAxis=[0 0 1]  FollAlignAxisA=+Z  BaseAlignAxisA=-Y  FollAlignAxisB=+X  BaseAlignAxisB=+X  RotationSequenceAxes=FollowerAxes  RotationSequence=ZYX  RotationSequenceAngles=[-90 0 90]  RotationSequenceAnglesUnits=deg  RotationMatrix=[1 0 0; 0 1 0; 0 0 1]
  Transform Axis4 : sm_lib/Frames and Transforms/Rigid Transform  TranslationMethod=Cartesian  TranslationStandardOffset=0  TranslationLengthUnit=mm  TranslationStandardAxis=+Z  TranslationCartesianOffset=[142 0 625]  TranslationROffset=0  TranslationROffsetUnits=m  TranslationZOffset=0  TranslationZOffsetUnits=m  TranslationThetaOffset=0  TranslationThetaOffsetUnits=deg  RotationMethod=RotationSequence  RotationAngleUnits=deg  RotationStandardAxis=+Z  RotationAngle=0.0  RotationArbitraryAxis=[0 0 1]  FollAlignAxisA=+Z  BaseAlignAxisA=+X  FollAlignAxisB=+X  BaseAlignAxisB=+Z  RotationSequenceAxes=FollowerAxes  RotationSequence=ZYX  RotationSequenceAngles=[0 -90 0]  RotationSequenceAnglesUnits=deg  RotationMatrix=[1 0 0; 0 1 0; 0 0 1]
  Transform Axis4-5 : sm_lib/Frames and Transforms/Rigid Transform  TranslationMethod=Cartesian  TranslationStandardOffset=0  TranslationLengthUnit=mm  TranslationStandardAxis=+Z  TranslationCartesianOffset=[0 0 -138]  TranslationROffset=0  TranslationROffsetUnits=m  TranslationZOffset=0  TranslationZOffsetUnits=m  TranslationThetaOffset=0  TranslationThetaOffsetUnits=deg  RotationMethod=RotationSequence  RotationAngleUnits=deg  RotationStandardAxis=+Z  RotationAngle=0.0  RotationArbitraryAxis=[0 0 1]  FollAlignAxisA=+Z  BaseAlignAxisA=+Y  FollAlignAxisB=+X  BaseAlignAxisB=+X  RotationSequenceAxes=FollowerAxes  RotationSequence=ZYX  RotationSequenceAngles=[90 90 0]  RotationSequenceAnglesUnits=deg  RotationMatrix=[1 0 0; 0 1 0; 0 0 1]
  Transform Axis5 : sm_lib/Frames and Transforms/Rigid Transform  TranslationMethod=Cartesian  TranslationStandardOffset=0  TranslationLengthUnit=mm  TranslationStandardAxis=+Z  TranslationCartesianOffset=[20+260 0 625]  TranslationROffset=0  TranslationROffsetUnits=m  TranslationZOffset=0  TranslationZOffsetUnits=m  TranslationThetaOffset=0  TranslationThetaOffsetUnits=deg  RotationMethod=RotationSequence  RotationAngleUnits=deg  RotationStandardAxis=+Z  RotationAngle=0.0  RotationArbitraryAxis=[0 0 1]  FollAlignAxisA=+Z  BaseAlignAxisA=-Y  FollAlignAxisB=+X  BaseAlignAxisB=+Z  RotationSequenceAxes=FollowerAxes  RotationSequence=ZYX  RotationSequenceAngles=[0 0 -90]  RotationSequenceAnglesUnits=deg  RotationMatrix=[1 0 0; 0 1 0; 0 0 1]
  Transform Axis5-1 : sm_lib/Frames and Transforms/Rigid Transform  TranslationMethod=Cartesian  TranslationStandardOffset=0  TranslationLengthUnit=mm  TranslationStandardAxis=+Z  TranslationCartesianOffset=[75 0 0]  TranslationROffset=0  TranslationROffsetUnits=m  TranslationZOffset=0  TranslationZOffsetUnits=m  TranslationThetaOffset=0  TranslationThetaOffsetUnits=deg  RotationMethod=RotationSequence  RotationAngleUnits=deg  RotationStandardAxis=+Z  RotationAngle=0.0  RotationArbitraryAxis=[0 0 1]  FollAlignAxisA=+Z  BaseAlignAxisA=-Y  FollAlignAxisB=-X  BaseAlignAxisB=+X  RotationSequenceAxes=FollowerAxes  RotationSequence=ZYX  RotationSequenceAngles=[-90 0 90]  RotationSequenceAnglesUnits=deg  RotationMatrix=[1 0 0; 0 1 0; 0 0 1]
  Transform Axis6 : sm_lib/Frames and Transforms/Rigid Transform  TranslationMethod=Cartesian  TranslationStandardOffset=0  TranslationLengthUnit=mm  TranslationStandardAxis=+Z  TranslationCartesianOffset=[20+260+75 0 625]  TranslationROffset=0  TranslationROffsetUnits=m  TranslationZOffset=0  TranslationZOffsetUnits=m  TranslationThetaOffset=0  TranslationThetaOffsetUnits=deg  RotationMethod=RotationSequence  RotationAngleUnits=deg  RotationStandardAxis=+Z  RotationAngle=0.0  RotationArbitraryAxis=[0 0 1]  FollAlignAxisA=+Z  BaseAlignAxisA=+X  FollAlignAxisB=-X  BaseAlignAxisB=+Z  RotationSequenceAxes=FollowerAxes  RotationSequence=ZYX  RotationSequenceAngles=[0 -90 0]  RotationSequenceAnglesUnits=deg  RotationMatrix=[1 0 0; 0 1 0; 0 0 1]
  Transform Ball : sm_lib/Frames and Transforms/Rigid Transform  TranslationMethod=None  TranslationStandardOffset=0  TranslationLengthUnit=mm  TranslationStandardAxis=+Z  TranslationCartesianOffset=[0 0 -80]  TranslationROffset=0  TranslationROffsetUnits=m  TranslationZOffset=0  TranslationZOffsetUnits=m  TranslationThetaOffset=0  TranslationThetaOffsetUnits=deg  RotationMethod=RotationSequence  RotationAngleUnits=deg  RotationStandardAxis=+Z  RotationAngle=0.0  RotationArbitraryAxis=[0 0 1]  FollAlignAxisA=+Z  BaseAlignAxisA=-Z  FollAlignAxisB=+X  BaseAlignAxisB=+Y  RotationSequenceAxes=FollowerAxes  RotationSequence=XYX  RotationSequenceAngles=[0 180 0]  RotationSequenceAnglesUnits=deg  RotationMatrix=[1 0 0; 0 1 0; 0 0 1]
  Transform Base-Axis1 : sm_lib/Frames and Transforms/Rigid Transform  TranslationMethod=StandardAxis  TranslationStandardOffset=183  TranslationLengthUnit=mm  TranslationStandardAxis=+Z  TranslationCartesianOffset=[0 0 183]  TranslationROffset=0  TranslationROffsetUnits=m  TranslationZOffset=0  TranslationZOffsetUnits=m  TranslationThetaOffset=0  TranslationThetaOffsetUnits=deg  RotationMethod=RotationSequence  RotationAngleUnits=deg  RotationStandardAxis=+Z  RotationAngle=0.0  RotationArbitraryAxis=[0 0 1]  FollAlignAxisA=+X  BaseAlignAxisA=+X  FollAlignAxisB=+Z  BaseAlignAxisB=+Z  RotationSequenceAxes=FollowerAxes  RotationSequence=ZYX  RotationSequenceAngles=[0 0 pi]  RotationSequenceAnglesUnits=rad  RotationMatrix=[1 0 0; 0 1 0; 0 0 1]
  Transform END : sm_lib/Frames and Transforms/Rigid Transform  TranslationMethod=Cartesian  TranslationStandardOffset=-40  TranslationLengthUnit=mm  TranslationStandardAxis=+Z  TranslationCartesianOffset=[0 0 34]  TranslationROffset=0  TranslationROffsetUnits=m  TranslationZOffset=0  TranslationZOffsetUnits=m  TranslationThetaOffset=0  TranslationThetaOffsetUnits=deg  RotationMethod=None  RotationAngleUnits=deg  RotationStandardAxis=+Z  RotationAngle=0.0  RotationArbitraryAxis=[0 0 1]  FollAlignAxisA=+Z  BaseAlignAxisA=+Z  FollAlignAxisB=+X  BaseAlignAxisB=+X  RotationSequenceAxes=FollowerAxes  RotationSequence=XYX  RotationSequenceAngles=[0 0 0]  RotationSequenceAnglesUnits=deg  RotationMatrix=[1 0 0; 0 1 0; 0 0 1]
  Transform offset1 : sm_lib/Frames and Transforms/Rigid Transform  TranslationMethod=None  TranslationStandardOffset=0  TranslationLengthUnit=mm  TranslationStandardAxis=+Z  TranslationCartesianOffset=[20 0 345]  TranslationROffset=0  TranslationROffsetUnits=m  TranslationZOffset=0  TranslationZOffsetUnits=m  TranslationThetaOffset=0  TranslationThetaOffsetUnits=deg  RotationMethod=RotationSequence  RotationAngleUnits=deg  RotationStandardAxis=-X  RotationAngle=90  RotationArbitraryAxis=[0 0 1]  FollAlignAxisA=+Z  BaseAlignAxisA=-Y  FollAlignAxisB=+X  BaseAlignAxisB=+X  RotationSequenceAxes=FollowerAxes  RotationSequence=ZYX  RotationSequenceAngles=[90 0 0]  RotationSequenceAnglesUnits=deg  RotationMatrix=[1 0 0; 0 1 0; 0 0 1]
  Transform offset2 : sm_lib/Frames and Transforms/Rigid Transform  TranslationMethod=None  TranslationStandardOffset=0  TranslationLengthUnit=mm  TranslationStandardAxis=+Z  TranslationCartesianOffset=[20 0 345]  TranslationROffset=0  TranslationROffsetUnits=m  TranslationZOffset=0  TranslationZOffsetUnits=m  TranslationThetaOffset=0  TranslationThetaOffsetUnits=deg  RotationMethod=RotationSequence  RotationAngleUnits=deg  RotationStandardAxis=-X  RotationAngle=90  RotationArbitraryAxis=[0 0 1]  FollAlignAxisA=+Z  BaseAlignAxisA=-Y  FollAlignAxisB=+X  BaseAlignAxisB=+X  RotationSequenceAxes=FollowerAxes  RotationSequence=ZYX  RotationSequenceAngles=[-90 0 0]  RotationSequenceAnglesUnits=deg  RotationMatrix=[1 0 0; 0 1 0; 0 0 1]
  World Frame : sm_lib/Frames and Transforms/World Frame
  rotmat2zyx-ang : Subsystem
  base : PMIOPort  Side=Left
  x : Outport  VectorParamsAs1DForOutWhenUnconnected=off
  y : Outport  Port=2  VectorParamsAs1DForOutWhenUnconnected=off
  z : Outport  Port=3  VectorParamsAs1DForOutWhenUnconnected=off
  rot : Outport  Port=4  VectorParamsAs1DForOutWhenUnconnected=off
  q_act : Outport  Port=5  VectorParamsAs1DForOutWhenUnconnected=off
  wires:
  Demux2/1 -> [q1]
  Demux2/5 -> [q5]
  [q1] -> Simulink-PS Converter7/1
  [q2] -> Simulink-PS Converter6/1
  [q3] -> Simulink-PS Converter8/1
  [q4] -> Simulink-PS Converter9/1
  [q5] -> Simulink-PS Converter10/1
  [q6] -> Simulink-PS Converter11/1
  PS-Simulink Converter2/1 -> y/1
  PS-Simulink Converter1/1 -> x/1
  PS-Simulink Converter3/1 -> z/1
  q/1 -> Demux2/1
  Demux2/4 -> [q4]
  Demux2/6 -> [q6]
  PS-Simulink Converter10/1 -> Mux/6
  PS-Simulink Converter9/1 -> Mux/5
  PS-Simulink Converter8/1 -> Mux/4
  PS-Simulink Converter5/1 -> Mux/1
  Mux/1 -> q_act/1
  Demux2/2 -> [q2]
  Demux2/3 -> [q3]
  PS-Simulink Converter6/1 -> Mux/2
  PS-Simulink Converter7/1 -> Mux/3
  PS-Simulink Converter4/1 -> rotmat2zyx-ang/1(rotmat)
  rotmat2zyx-ang/1(zyx-ang) -> rot/1
  connections:
  Axis1/RConn1 -- Transform Axis1/LConn1
  " Joint q1"/LConn1 -- Transform Base-Axis1/RConn1
  Transform Axis1/RConn1 -- Transform Axis1-2/LConn1 -- " Joint q1"/RConn1
  " Joint q2"/LConn1 -- Transform Axis1-2/RConn1
  Axis2/RConn1 -- Transform Axis2/LConn1
  " Joint q4"/RConn1 -- Transform Axis4/RConn1 -- Transform Axis4-5/LConn1
  Transform Axis3/LConn1 -- Axis3/RConn1
  " Joint q3"/LConn1 -- Transform Axis2-3/RConn1
  Transform Axis4/LConn1 -- Axis4/RConn1
  " Joint q4"/LConn1 -- Transform Axis3-4/RConn1
  Transform Axis4-5/RConn1 -- " Joint q5"/LConn1
  Transform Axis5/LConn1 -- Axis5/RConn1
  Transform Axis5-1/RConn1 -- " Joint q6"/LConn1
  Transform Axis6/LConn1 -- Axis6/RConn1
  " Joint q1"/LConn2 -- PS Gain6/RConn1
  PS Gain4/RConn1 -- " Joint q3"/LConn2
  PS Gain3/RConn1 -- " Joint q6"/LConn2
  PS Gain1/RConn1 -- " Joint q5"/LConn2
  PS Gain2/RConn1 -- " Joint q4"/LConn2
  PS Gain5/RConn1 -- " Joint q2"/LConn2
  Transform Sensor/RConn1 -- Transform END/LConn1 -- Transform Ball/RConn1
  Mechanism Configuration/RConn1 -- Transform Sensor/LConn1 -- Transform Base-Axis1/LConn1 -- Base/RConn1 -- base/RConn1 -- Solver Configuration/RConn1 -- World Frame/RConn1
  Axis7/RConn1 -- Transform END/RConn1
  Transform Axis2-3/LConn1 -- Transform offset2/RConn1 -- " Joint q2"/RConn1
  Transform Axis3-4/LConn1 -- Transform offset1/RConn1 -- " Joint q3"/RConn1
  Transform Axis5-1/LConn1 -- Transform Axis5/RConn1 -- " Joint q5"/RConn1
  " Joint q6"/RConn1 -- Transform Axis6/RConn1 -- Transform Ball/LConn1
  Transform Sensor/RConn2 -- PS-Simulink Converter4/LConn1
  " Joint q1"/RConn2 -- PS-Simulink Converter5/LConn1
  " Joint q2"/RConn2 -- PS-Simulink Converter6/LConn1
  " Joint q3"/RConn2 -- PS-Simulink Converter7/LConn1
  " Joint q4"/RConn2 -- PS-Simulink Converter8/LConn1
  " Joint q5"/RConn2 -- PS-Simulink Converter9/LConn1
  " Joint q6"/RConn2 -- PS-Simulink Converter10/LConn1
  Simulink-PS Converter7/RConn1 -- PS Gain6/LConn1
  Simulink-PS Converter6/RConn1 -- PS Gain5/LConn1
  Simulink-PS Converter8/RConn1 -- PS Gain4/LConn1
  Simulink-PS Converter9/RConn1 -- PS Gain2/LConn1
  Simulink-PS Converter10/RConn1 -- PS Gain1/LConn1
  Simulink-PS Converter11/RConn1 -- PS Gain3/LConn1
  Transform offset2/LConn1 -- Transform Axis2/RConn1
  Transform offset1/LConn1 -- Transform Axis3/RConn1
  Transform Sensor/RConn3 -- PS-Simulink Converter1/LConn1
  Transform Sensor/RConn4 -- PS-Simulink Converter2/LConn1
  Transform Sensor/RConn5 -- PS-Simulink Converter3/LConn1

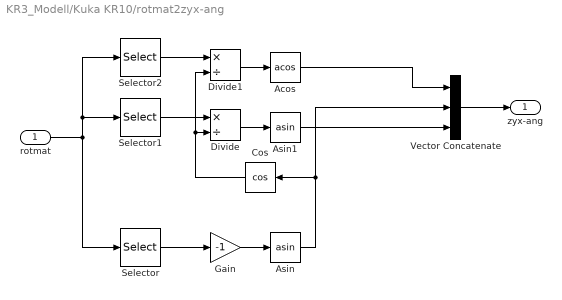
== system KR3_Modell/Kuka KR10/rotmat2zyx-ang ==
  rotmat : Inport
  Acos : Trigonometry  Operator=acos
  Asin : Trigonometry  Operator=asin
  Asin1 : Trigonometry  Operator=asin
  Cos : Trigonometry  Operator=cos
  Divide : Product  Inputs=*/
  Divide1 : Product  Inputs=*/
  Gain : Gain  Gain=-1
  Selector : Selector  NumberOfDimensions=2  InputPortWidth=3  IndexOptions=Index vector (dialog),Index vector (dialog)  Indices=3,1  OutputSizes=1,1
  Selector1 : Selector  NumberOfDimensions=2  InputPortWidth=3  IndexOptions=Index vector (dialog),Index vector (dialog)  Indices=3,2  OutputSizes=1,1
  Selector2 : Selector  NumberOfDimensions=2  InputPortWidth=3  IndexOptions=Index vector (dialog),Index vector (dialog)  Indices=1,1  OutputSizes=1,1
  Vector Concatenate : Concatenate  NumInputs=3
  zyx-ang : Outport
  wires:
  Cos/1 -> Divide1/2, Divide/2
  Divide/1 -> Asin1/1
  Selector1/1 -> Divide/1
  Asin/1 -> Vector Concatenate/2, Cos/1
  Acos/1 -> Vector Concatenate/1
  Vector Concatenate/1 -> zyx-ang/1
  Gain/1 -> Asin/1
  Divide1/1 -> Acos/1
  rotmat/1 -> Selector2/1, Selector1/1, Selector/1
  Asin1/1 -> Vector Concatenate/3
  Selector/1 -> Gain/1
  Selector2/1 -> Divide1/1

== matlab function KR3_Modell/Position and angle to transform homogeneous matrix1 ==
  data: xyz input; T output; abc input
function T = posang2transmat(xyz,abc)

a=abc(1)*pi/180;
b=abc(2)*pi/180;
c=abc(3)*pi/180;


Rx=[ 1, 0, 0;
     0, cos(c), -sin(c);
     0, sin(c), cos(c)];

Ry=[cos(b)  0, sin(b);
     0     1,      0;
  -sin(b), 0, cos(b)];

Rz=[cos(a), -sin(a), 0;
   sin(a),  cos(a), 0;
        0,       0, 1];
    

T=[[Rz*Ry*Rx; [0 0 0]], [reshape(xyz,3,1); 1]];
